simulink model "single_track_v2"  (R2024a)
settings: Solver=VariableStepAuto  StartTime=0.0  StopTime=145  RelTol=1e-3
undefined symbols (not defined in the file or in its folder): control_param, veh_param
libraries: simulink x5, autolibshared x1
settings Model: Creator=pair-andres  LastModifiedBy=pair-andres

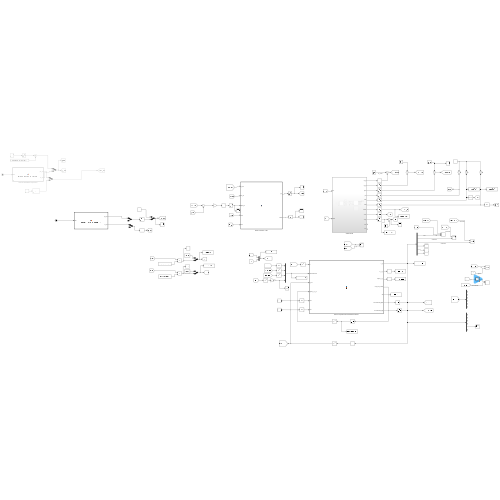
[thumbnail: Simulink's stored preview of the top-level diagram]
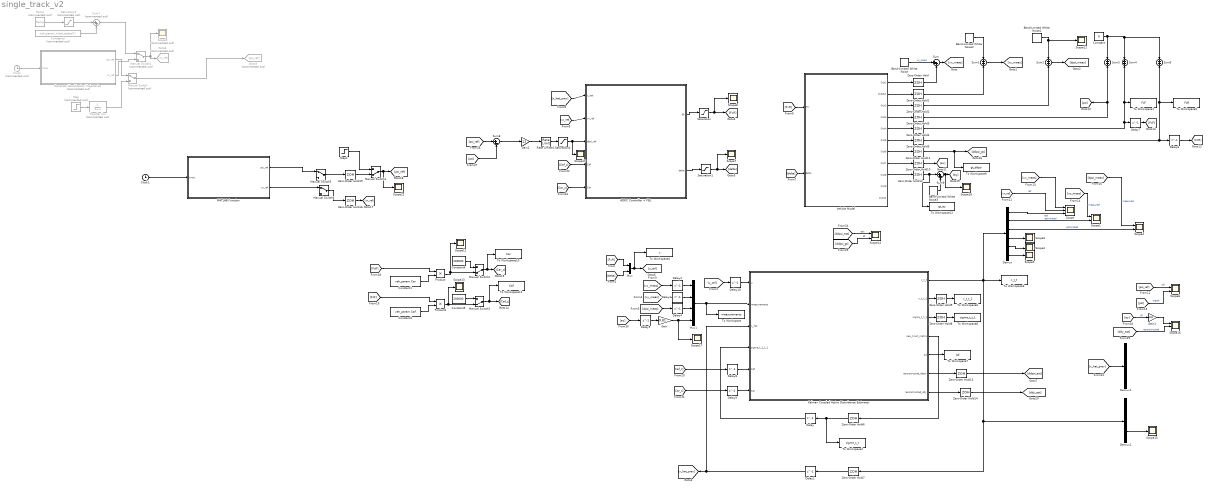
== system single_track_v2 ==
  ADRC Controller + FBL : MATLAB Function  TreatAsAtomicUnit=on
  Band-Limited White Noise : simulink/Sources/Band-Limited White Noise  Cov=[control_param.vx_noise_pwr]  Ts=control_param.T  seed=[23341]
  Band-Limited White Noise1 : simulink/Sources/Band-Limited White Noise  Cov=[control_param.dpsi_noise_pwr]  Ts=control_param.T  seed=[23343]
  Band-Limited White Noise2 : simulink/Sources/Band-Limited White Noise  Cov=[control_param.vy_noise_pwr]  Ts=control_param.T  seed=[23342]
  Band-Limited White Noise3 : simulink/Sources/Band-Limited White Noise  Cov=[control_param.dpsi_noise_pwr]  Ts=control_param.T  seed=[23343]
  Clock : Clock  Commented=on
  Clock1 : Clock
  Constant : Constant  Value=0
  Constant1 : Constant  Value=veh_param.Car  SampleTime=control_param.T
  Constant2 : Constant  Value=veh_param.Caf  SampleTime=control_param.T
  Constant3 : Constant  Commented=on  Value=veh_param.initial_states(1)
  Constant4 : Constant  Value=200000
  Constant5 : Constant  Value=200000
  Delay : Delay  DelayLength=1  InitialCondition=eye(6)*0  SampleTime=control_param.T
  Delay1 : Delay  DelayLength=1  InitialCondition=veh_param.initial_states  SampleTime=control_param.T
  Delay{2..5,8..10} (7 alike) : Delay  DelayLength=1  InitialCondition=0  SampleTime=control_param.T
  Delay6 : Delay  DelayLength=1  InitialCondition=veh_param.initial_states(1)  SampleTime=control_param.T
  Delay7 : Delay  DelayLength=1  InitialCondition=veh_param.initial_states(1)  SampleTime=control_param.T
  Demux : Demux  Outputs=6
  Demux1 : Demux  Outputs=6
  Demux2 : Demux  Outputs=6
  Gain : Gain  Gain=9.81
  Gain1 : Gain  Gain=9.81
  Gain2 : Gain  Gain=12
  Generate Identification Trajectories : MATLAB Function  Commented=on  TreatAsAtomicUnit=on
  Goto8 : Goto  Commented=on  GotoTag=vx_ref
  Goto9 : Goto  Commented=on  GotoTag=psi_ref
  Kalman Coupled Active Disturbance Estimator : MATLAB Function  TreatAsAtomicUnit=on
  MATLAB Function : MATLAB Function  TreatAsAtomicUnit=on
  Manual Switch : ManualSwitch  Commented=on
  Manual Switch1 : ManualSwitch  Commented=on
  Manual Switch2 : ManualSwitch  CurrentSetting=0
  Manual Switch3 : ManualSwitch  CurrentSetting=0
  Manual Switch4 : ManualSwitch  CurrentSetting=0
  Manual Switch5 : ManualSwitch
  Manual Switch6 : ManualSwitch
  Mux : Mux  Inputs=2
  Mux1 : Mux
  Product : Product
  Product1 : Product
  Ramp : simulink/Sources/Ramp  Commented=on  slope=5  start=2  InitialOutput=5
  Rate Limiter1 : RateLimiter  RisingSlewLimit=1.0  FallingSlewLimit=-1.0  SampleTimeMode=inherited
  Saturation : Saturate  UpperLimit=2000  LowerLimit=-4000
  Saturation1 : Saturate  UpperLimit=0.262  LowerLimit=-0.262
  Saturation2 : Saturate  Commented=on  UpperLimit=30
  Saturation4 : Saturate  UpperLimit=0.3  LowerLimit=-0.3
  Scope : Scope  NumInputPorts=3
  Scope{1..2,6,14} (4 alike) : Scope  NumInputPorts=2
  Scope{3..5,7..8,10..13,15,17..18,22} (13 alike) : Scope
  Scope16 : Scope  NumInputPorts=3
  Scope9 : Scope  Commented=on
  Step : Step  Commented=on  Time=5  After=0.1  SampleTime=0
  Step1 : Step  Time=0  After=0.05  SampleTime=control_param.T
  Sum : Sum  Inputs=|++
  Sum{1..5} (5 alike) : Sum
  Sum7 : Sum  Commented=on  Inputs=|++
  Sum8 : Sum  Inputs=|+-
  Sum9 : Sum  Inputs=|++
  To Workspace : ToWorkspace  VariableName=measurements  SaveFormat=Timeseries  SampleTime=control_param.T
  To Workspace1 : ToWorkspace  VariableName=FzF  SaveFormat=Timeseries  SampleTime=control_param.T
  To Workspace10 : ToWorkspace  VariableName=Car  SaveFormat=Timeseries  SampleTime=control_param.T
  To Workspace11 : ToWorkspace  VariableName=Caf  SaveFormat=Timeseries  SampleTime=control_param.T
  To Workspace12 : ToWorkspace  VariableName=gt_ay  SaveFormat=Timeseries  SampleTime=control_param.T
  To Workspace2 : ToWorkspace  VariableName=sigma_t_t  SaveFormat=Timeseries  SampleTime=0.01
      settings: Save2DSignal=2-D array (concatenate along first dimension)
  To Workspace3 : ToWorkspace  VariableName=x_t_t  SaveFormat=Timeseries  SampleTime=control_param.T
  To Workspace4 : ToWorkspace  VariableName=u  SaveFormat=Timeseries  SampleTime=control_param.T
  To Workspace5 : ToWorkspace  VariableName=FzR  SaveFormat=Timeseries  SampleTime=control_param.T
  To Workspace6 : ToWorkspace  VariableName=x_t_t_1  SaveFormat=Timeseries  SampleTime=0.01
  To Workspace7 : ToWorkspace  VariableName=Ad  SaveFormat=Timeseries  SampleTime=control_param.T
  To Workspace8 : ToWorkspace  VariableName=sigma_t_t_1  SaveFormat=Timeseries  SampleTime=0.01
      settings: Save2DSignal=2-D array (concatenate along first dimension)
  To Workspace9 : ToWorkspace  VariableName=gt_ddpsi  SaveFormat=Timeseries  SampleTime=control_param.T
  Transfer Fcn : TransferFcn  Commented=on  Denominator=[1 1]
  Vehicle Model : Subsystem
  Zero-Order Hold{,1..16} (17 alike) : ZeroOrderHold  SampleTime=control_param.T
  wires:
  Vehicle Model/2(Output) -> Zero-Order Hold1/1
  Constant/1 -> Sum5/1, Sum4/1, Sum3/1
  Sum/1 -> [vx_meas]
  Band-Limited White Noise2/1 -> Sum1/1
  Zero-Order Hold3/1 -> [psi], Sum3/2
  Zero-Order Hold4/1 -> Delay7/1, To Workspace1/1, Sum4/2
  Sum2/1 -> [dpsi_meas]
  Zero-Order Hold6/1 -> To Workspace2/1, Delay/1
  Band-Limited White Noise/1 -> Sum/1  "vx_noise"
  Zero-Order Hold1/1 -> Sum1/2
  Vehicle Model/6(Out5) -> Zero-Order Hold5/1
  Band-Limited White Noise1/1 -> Scope11/1, Sum2/1
  Vehicle Model/5(Out4) -> Zero-Order Hold4/1
  Delay/1 -> Kalman Coupled Active Disturbance Estimator/4(sigma_t_1_t_1)
  Vehicle Model/4(Out3) -> Zero-Order Hold3/1
  Vehicle Model/1(Out1) -> Zero-Order Hold/1
  Zero-Order Hold2/1 -> Sum2/2
  Vehicle Model/3(Out2) -> Zero-Order Hold2/1
  Sum1/1 -> [vy_meas]
  Zero-Order Hold/1 -> Sum/2
  Zero-Order Hold5/1 -> Delay6/1, To Workspace5/1, Sum5/2
  Kalman Coupled Active Disturbance Estimator/5(Ad) -> To Workspace7/1
  Kalman Coupled Active Disturbance Estimator/1(x_t_t) -> Demux2/1, Zero-Order Hold7/1, To Workspace3/1, Demux/1
  Zero-Order Hold7/1 -> Delay1/1
  Delay1/1 -> [x_hat_prev], Kalman Coupled Active Disturbance Estimator/3(x_hat)
  ADRC Controller + FBL/1(gp) -> Saturation/1
  ADRC Controller + FBL/2(delta) -> Saturation1/1
  [FxR] -> Mux/1
  [delta] -> Mux/2
  Mux/1 -> To Workspace4/1, [u_ctrl]
  Kalman Coupled Active Disturbance Estimator/2(x_t_t_1) -> Zero-Order Hold9/1
  Zero-Order Hold9/1 -> To Workspace6/1
  [u_ctrl] -> Delay10/1
  [dpsi_meas] -> Delay4/1
  [vx_meas] -> Delay2/1
  Mux1/1 -> To Workspace/1, Kalman Coupled Active Disturbance Estimator/2(measurements)
  [delta] -> Vehicle Model/2(delta)
  [FxR] -> Vehicle Model/1(Fxr)
  Kalman Coupled Active Disturbance Estimator/3(sigma_t_t_1) -> Zero-Order Hold8/1
  Zero-Order Hold8/1 -> To Workspace8/1
  Kalman Coupled Active Disturbance Estimator/4(new_trust_matrix) -> Zero-Order Hold6/1
  Kalman Coupled Active Disturbance Estimator/6(reconstructed_ddpsi) -> Zero-Order Hold13/1
  [x_hat_prev] -> ADRC Controller + FBL/1(x_hat)
  Clock/1 -> Generate Identification Trajectories/1(time)
  Demux/6 -> Scope5/1
  Demux/5 -> Scope4/1
  Demux/4 -> Scope3/1
  Demux/3 -> Scope2/2  "estimated"
  Demux/2 -> Scope1/2  "estimated"
  Demux/1 -> Scope/3  "est"
  [vx_ref] -> ADRC Controller + FBL/2(vx_ref)
  [vx_ref] -> Scope/2  "ref"
  Saturation/1 -> Scope8/1, [FxR]
  Saturation1/1 -> Scope7/1, [delta]
  [vx_meas] -> Scope/1
  [vy_meas] -> Scope1/1  "measured"
  Generate Identification Trajectories/1(psi_ref) -> Manual Switch/1
  Manual Switch/1 -> Goto9/1
  [psi_ref] -> Scope6/1  "ref"
  [psi] -> Scope6/2  "signal"
  [dpsi_meas] -> Scope2/1  "measured"
  Vehicle Model/8(Out7) -> Zero-Order Hold10/1
  Zero-Order Hold10/1 -> [ax]
  Step/1 -> Transfer Fcn/1
  Generate Identification Trajectories/2(vx_ref) -> Manual Switch1/2
  Manual Switch1/1 -> Goto8/1, Scope9/1
  Constant1/1 -> Product/2
  Constant2/1 -> Product1/2
  Product/1 -> Manual Switch2/2, Scope12/1
  Product1/1 -> Manual Switch3/2, Scope13/1
  [Car_z] -> Delay9/1
  [Caf_z] -> Delay8/1
  [Caf_z] -> ADRC Controller + FBL/4(Caf)
  [Car_z] -> ADRC Controller + FBL/5(Car)
  Ramp/1 -> Saturation2/1
  Constant3/1 -> Sum7/2
  Sum7/1 -> Manual Switch1/1
  Saturation2/1 -> Sum7/1
  [FzR] -> Product/1
  [FzF] -> Product1/1
  Vehicle Model/7(Out6) -> Zero-Order Hold11/1
  Zero-Order Hold11/1 -> To Workspace9/1, [ddpsi_gt]
  [ddpsi_est] -> Scope14/1  "est"
  [ddpsi_gt] -> Scope14/2  "gt"
  Constant4/1 -> Manual Switch2/1
  Constant5/1 -> Manual Switch3/1
  Transfer Fcn/1 -> Manual Switch/2
  Manual Switch2/1 -> To Workspace10/1, [Car_z]
  Manual Switch3/1 -> To Workspace11/1, [Caf_z]
  Step1/1 -> Manual Switch4/1
  Clock1/1 -> MATLAB Function/1(time)
  Manual Switch4/1 -> Scope22/1, [psi_ref]
  Gain2/1 -> Rate Limiter1/1
  Rate Limiter1/1 -> Saturation4/1
  [psi] -> Sum8/2
  [psi_ref] -> Sum8/1
  Saturation4/1 -> Scope10/1, ADRC Controller + FBL/3(dpsi_ref)
  Delay6/1 -> [FzR]
  Delay7/1 -> [FzF]
  [vy_meas] -> Delay3/1
  Vehicle Model/9(Out8) -> Zero-Order Hold12/1
  Kalman Coupled Active Disturbance Estimator/7(reconstructed_ddy) -> Zero-Order Hold14/1
  [ay] -> Gain1/1  "gt"
  [ddy_est] -> Scope16/2  "reconstructed"
  [ay] -> Delay5/1
  Zero-Order Hold12/1 -> To Workspace12/1, Sum9/1
  Band-Limited White Noise3/1 -> Sum9/2
  Sum9/1 -> Scope18/1, [ay]
  Sum8/1 -> Gain2/1
  Zero-Order Hold13/1 -> [ddpsi_est]
  Zero-Order Hold14/1 -> [ddy_est]
  [x_hat_prev] -> Demux1/1
  Delay2/1 -> Mux1/1
  Delay3/1 -> Mux1/2
  Delay4/1 -> Mux1/3
  Delay5/1 -> Gain/1
  Delay8/1 -> Kalman Coupled Active Disturbance Estimator/5(Caf)
  Delay9/1 -> Kalman Coupled Active Disturbance Estimator/6(Car)
  Delay10/1 -> Kalman Coupled Active Disturbance Estimator/1(u)
  Zero-Order Hold15/1 -> Manual Switch4/2
  Zero-Order Hold16/1 -> [vx_ref]
  Manual Switch5/1 -> Zero-Order Hold15/1
  MATLAB Function/1(psi_ref) -> Manual Switch5/1
  Manual Switch6/1 -> Zero-Order Hold16/1
  MATLAB Function/2(vx_ref) -> Manual Switch6/1
  Gain/1 -> Scope17/1, Mux1/4
  Demux2/5 -> Scope15/1
  Gain1/1 -> Scope16/1

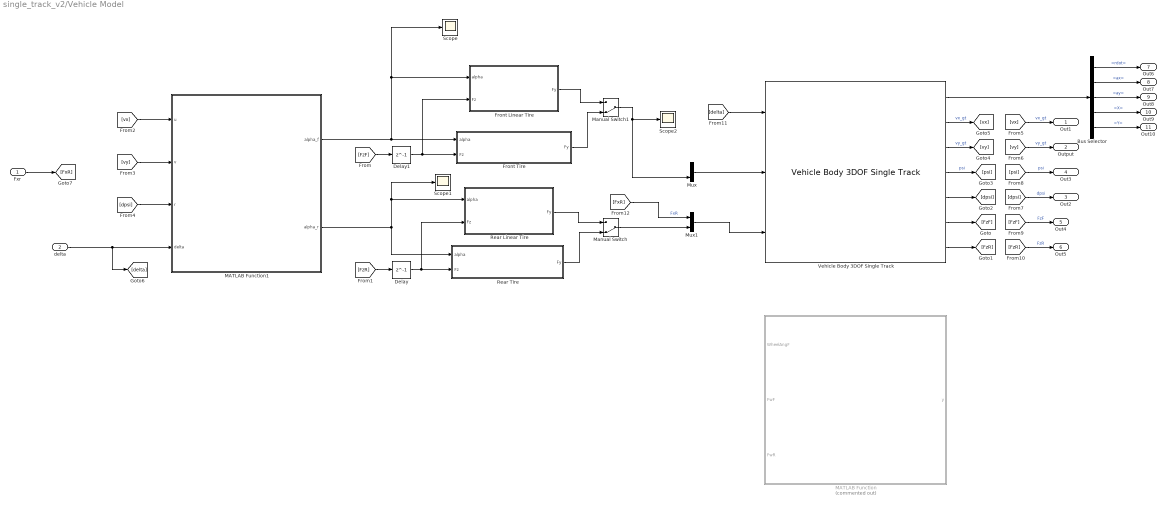
== system single_track_v2/Vehicle Model ==
  Fxr : Inport
  delta : Inport  Port=2
  Bus Selector : BusSelector  OutputSignals=BdyFrm.Cg.AngAcc.rdot,BdyFrm.Cg.Acc.ax,BdyFrm.Cg.Acc.ay,InertFrm.Cg.Disp.X,InertFrm.Cg.Disp.Y
  Delay : Delay  DelayLength=1  InitialCondition=veh_param.m*veh_param.g / 2  SampleTime=control_param.T
  Delay1 : Delay  DelayLength=1  InitialCondition=veh_param.m*veh_param.g / 2  SampleTime=control_param.T
  Front Linear Tire : MATLAB Function  TreatAsAtomicUnit=on
  Front Tire : MATLAB Function  TreatAsAtomicUnit=on
  MATLAB Function : MATLAB Function  Commented=on  TreatAsAtomicUnit=on
  MATLAB Function1 : MATLAB Function  TreatAsAtomicUnit=on
  Manual Switch : ManualSwitch  CurrentSetting=0
  Manual Switch1 : ManualSwitch  CurrentSetting=0
  Mux : Mux  Inputs=2
  Mux1 : Mux  Inputs=2
  Rear Linear Tire : MATLAB Function  TreatAsAtomicUnit=on
  Rear Tire : MATLAB Function  TreatAsAtomicUnit=on
  Scope : Scope
  Scope1 : Scope
  Scope2 : Scope
  Vehicle Body 3DOF Single Track : autolibshared/Vehicle Body 3DOF Single Track  trackMode=Single (bicycle)  inputMode=External forces  frontSteerMode=on  rearSteerMode=off  windMode=off  muMode=off  extFMode=off  extMMode=off  htchFMode=off  htchMMode=off  extXo=off  extpsio=off  extxdoto=off  extro=off  extYo=off  extTamb=off  extydoto=off  aMode=2  NF=2  NR=2  m=veh_param.m  a=veh_param.lf  b=veh_param.lr  h=0.35  dh=1  hh=0.2  X_o=0  xdot_o=veh_param.initial_states(1)  CalphaMode=off  sigmaMode=on  d=0  hl=0  w=[1.4,1.4]  Cy_f=12e3  Cy_r=11e3  sigma_f=.1  sigma_r=.1  alpha_f_brk=[-.1 .1]  Cy_f_data=[-9e3 9e3]  alpha_r_brk=[-.1 .1]  Cy_r_data=[-9e3 9e3]  Y_o=500  ydot_o=0  Izz=1000  psi_o=0  r_o=0  Af=2.0  Cd=veh_param.Cd  Cl=.1  Cpm=.1  beta_w=[0 0.01:0.01:0.3]  Cs=[0 0.01:0.01:0.3]  Cym=[0 1e-6:0.01:0.3]  Pabs=101325  Tair=273  g=9.81  mu=1  xdot_tol=.01  Fznom=5000  Fxtire_sat=7e4  Fytire_sat=7e4  longOff=0  latOff=0  vertOff=0  wrapAng=off
  Out1 : Outport
  Output : Outport  Port=2
  Out2 : Outport  Port=3
  Out3 : Outport  Port=4
  Out4 : Outport  Port=5
  Out5 : Outport  Port=6
  Out6 : Outport  Port=7
  Out7 : Outport  Port=8
  Out8 : Outport  Port=9
  Out9 : Outport  Port=10
  Out10 : Outport  Port=11
  wires:
  Bus Selector/5 -> Out10/1  "<Y>"
  Bus Selector/2 -> Out7/1  "<ax>"
  [FzF] -> Delay1/1
  Vehicle Body 3DOF Single Track/3 -> [vy]  "vy_gt"
  Mux/1 -> Vehicle Body 3DOF Single Track/2
  Vehicle Body 3DOF Single Track/1 -> Bus Selector/1
  Bus Selector/1 -> Out6/1  "<rdot>"
  [FzR] -> Out5/1  "FzR"
  Vehicle Body 3DOF Single Track/4 -> [psi]  "psi"
  [vx] -> MATLAB Function1/1(u)
  Fxr/1 -> [FxR]
  MATLAB Function1/2(alpha_r) -> Scope1/1, Rear Linear Tire/1(alpha), Rear Tire/1(alpha)
  Vehicle Body 3DOF Single Track/7 -> [FzR]
  Rear Linear Tire/1(Fy) -> Manual Switch/1
  [FzR] -> Delay/1
  Vehicle Body 3DOF Single Track/5 -> [dpsi]
  MATLAB Function1/1(alpha_f) -> Scope/1, Front Linear Tire/1(alpha), Front Tire/1(alpha)
  Bus Selector/4 -> Out9/1  "<X>"
  Vehicle Body 3DOF Single Track/6 -> [FzF]
  Vehicle Body 3DOF Single Track/2 -> [vx]  "vx_gt"
  [vy] -> MATLAB Function1/2(v)
  [dpsi] -> Out2/1  "dpsi"
  Mux1/1 -> Vehicle Body 3DOF Single Track/3
  [delta] -> Vehicle Body 3DOF Single Track/1
  delta/1 -> [delta], MATLAB Function1/4(delta)
  Rear Tire/1(Fy) -> Manual Switch/2
  Front Tire/1(Fy) -> Manual Switch1/2
  Front Linear Tire/1(Fy) -> Manual Switch1/1
  [dpsi] -> MATLAB Function1/3(r)
  Bus Selector/3 -> Out8/1  "<ay>"
  [FxR] -> Mux1/1  "FxR"
  [psi] -> Out3/1  "psi"
  [FzF] -> Out4/1  "FzF"
  [vx] -> Out1/1  "vx_gt"
  [vy] -> Output/1  "vy_gt"
  Delay/1 -> Rear Linear Tire/2(Fz), Rear Tire/2(Fz)
  Delay1/1 -> Front Linear Tire/2(Fz), Front Tire/2(Fz)
  Manual Switch/1 -> Mux1/2
  Manual Switch1/1 -> Scope2/1, Mux/2

== matlab function single_track_v2/Vehicle Model/MATLAB Function1 ==
  data: u input; alpha_f output; v input; r input; delta input; alpha_r output; veh_param parameter
function [alpha_f, alpha_r] = calc_bicycle_slip_angles(u, v, r, delta, veh_param)
% Calculate slip angles at the tires:
% WARNING: Careful with sign conventions used in the model, make sure you
% get this right

lf = veh_param.lf;
lr = veh_param.lr;


theta_v_f = atan2(v + r * lf, u);

theta_v_r = atan2(v - r * lr, u);

% Front: Steer angle is delta, velocity angle is theta_v_f
alpha_f = theta_v_f - delta;

% Rear: Steer angle is 0, velocity angle is theta_v_r
alpha_r = theta_v_r;

end

== matlab function single_track_v2/Vehicle Model/Rear Linear Tire ==
  data: alpha input; Fy output; Fz input; veh_param parameter
function Fy = linear_tire_model(alpha, Fz, veh_param)
    % Implements a simple LINEAR tire model.
    %
    % Fy = C_alpha * alpha
    %
    % To be a fair comparison to your Pacejka block, we define
    % C_alpha as the initial slope of the Pacejka curve, which
    % is load-dependent.
    
    % TIRE PACEJKA PARAMS:
    B = veh_param.Br;
    C = veh_param.Cr;
    D = veh_param.Dr;
    E = veh_param.Er;
    
    % The linear cornering stiffness (C_alpha) for small angles
    % is the product of B, C, and D, scaled by Fz.
    % K is the "cornering stiffness coefficient".
    K_pacejka = B * C * D; % 22 * 1.8 * 1.6 = 63.36
    
    % --- Safety Check: Ensure Fz is positive ---
    Fz_pos = max(0, Fz);
    
    % --- 1. Calculate Cornering Stiffness ---
    C_alpha = K_pacejka * Fz_pos; % K * Fz_pos;
    
    % --- 2. Linear Force Calculation ---
    Fy = C_alpha * alpha;
end

== matlab function single_track_v2/Vehicle Model/Rear Tire ==
  data: alpha input; Fy output; Fz input; veh_param parameter
function Fy = simple_pacejka_lat(alpha, Fz, veh_param)

    % Implements the simple Pacejka '89 lateral force model.
    %
    % INPUTS:
    %   alpha:  Tire Slip Angle (radians)
    %   Fz:     Vertical Load on the tire (Newtons)
    %
    % OUTPUT:
    %   Fy:     Lateral Force (Newtons)
    
    % TIRE PACEJKA PARAMS:
    %   B:      Stiffness Factor
    %   C:      Shape Factor
    %   D:      Peak Factor (Peak friction coefficient, mu_y)
    %   E:      Curvature Factor
       
    % Front tire pacejka parameters:
    B = veh_param.Br;
    C = veh_param.Cr;
    D = veh_param.Dr;
    E = veh_param.Er;
    
    % --- Safety Check: Ensure Fz is positive ---
    % The formula assumes positive vertical load.
    Fz_pos = max(0, Fz);
    
    % --- 1. Calculate Peak Lateral Force ---
    % D is the friction coefficient, so F_peak = D * Fz
    F_peak = D * Fz_pos;
    
    % --- 2. Composite Slip Term ---
    % This is the main input to the sine function
    x = B * alpha;
    
    % --- 3. Pacejka '89 "Magic Formula" ---
    % This is the core equation
    Fy = -F_peak * sin(C * atan(x - E * (x - atan(x))));

end

== matlab function single_track_v2/Generate Identification Trajectories ==
  data: psi_ref output; vx_ref output; time input
function [psi_ref, vx_ref] = generate_identification_trajectory(time)
%#codegen
% Generates feasible, persistently exciting reference signals for 
% Vehicle System Identification.
%
% INPUT:
%   time: Current simulation time (seconds)
%
% OUTPUTS:
%   psi_ref: Global heading reference (radians)
%   vx_ref:  Longitudinal velocity reference (m/s) [10 to 40 m/s]
    

    % --- CONFIGURATION ---
    TEST_DURATION = 150; % Total test time (seconds)
    
    % Velocity Constraints
    V_MIN = 10; % m/s
    V_MAX = 40; % m/s
    
    % Heading Chirp Parameters
    % We want to sweep from gentle turns to aggressive slalom
    FREQ_START = 0.1; % Hz (Slow turns)
    FREQ_END   = 0.8; % Hz (Fast slalom - verify your sampling rate > 2*FREQ_END)
    AMP_YAW    = 0.1; % rad (Approx 30 degrees max heading deviation)

    % --- 1. GENERATE VELOCITY REFERENCE (vx_ref) ---
    % We use a slow sine wave to sweep through the speed range.
    % This ensures we test high-speed/low-steer and low-speed/high-steer.
    
    % Period of speed change (make it slower than steering dynamics)
    v_period = 10; 
    
    % Sine wave scaled to [V_MIN, V_MAX]
    % 0.5*(Max-Min)*sin(...) + 0.5*(Max+Min)
    vx_ref = 0.5 * (V_MAX - V_MIN) * sin(2 * pi * (1/v_period) * time - pi/2) ...
           + 0.5 * (V_MAX + V_MIN);
       
    % Clamp for safety (redundant but good practice)
    if vx_ref < V_MIN; vx_ref = V_MIN; end
    if vx_ref > V_MAX; vx_ref = V_MAX; end

    % --- 2. GENERATE HEADING REFERENCE (psi_ref) ---
    % We use a "Chirp" signal (Swept Sine) for the heading.
    % Ideally, we want the yaw rate to be the chirp, so psi is the integral.
    
    if time < 10
        % Stop the test
        psi_ref = 0;
        vx_ref = 5;

    elseif time <= TEST_DURATION
        % Instantaneous frequency f(t) = f0 + k*t
        k = (FREQ_END - FREQ_START) / TEST_DURATION;
        
        % Phase = integral of frequency
        % phi(t) = 2*pi * (f0*t + 0.5*k*t^2)
        phase = 2 * pi * (FREQ_START * time + 0.5 * k * time^2*0.2);
        
        % We modulate the amplitude based on speed to keep lateral accel safe-ish.
        % At 40 m/s, we can't turn as sharp as at 10 m/s.
        % Scaling factor: inversely proportional to speed
        safe_scaling = (V_MIN / vx_ref); 
        
        % The Heading Reference
        psi_ref = (AMP_YAW * safe_scaling) * sin(phase);
    else
        psi_ref = 0;
        vx_ref = 0;
    end
end

== matlab function single_track_v2/MATLAB Function ==
  data: time input; psi_ref output; vx_ref output
function [psi_ref, vx_ref] = generate_identification_trajectory(time)
%#codegen
% Generates feasible, persistently exciting reference signals for 
% Vehicle System Identification.
%
% INPUT:
%   time: Current simulation time (seconds)
%
% OUTPUTS:
%   psi_ref: Global heading reference (radians)
%   vx_ref:  Longitudinal velocity reference (m/s) [10 to 40 m/s]

    % --- CONFIGURATION ---
    TEST_DURATION = 150; % Total test time (seconds)
    
    % Velocity Constraints
    V_MIN = 10; % m/s
    V_MAX = 80; % m/s
    
    % Heading Chirp Parameters
    % We want to sweep from gentle turns to aggressive slalom
    FREQ_START = 0.001; % Hz (Slow turns)
    FREQ_END   = 0.8; % Hz (Fast slalom - verify your sampling rate > 2*FREQ_END)
    AMP_YAW    = 0.35; % rad (Approx 30 degrees max heading deviation)

    % --- 1. GENERATE VELOCITY REFERENCE (vx_ref) ---
    % We use a slow sine wave to sweep through the speed range.
    % This ensures we test high-speed/low-steer and low-speed/high-steer.
    
    % Period of speed change (make it slower than steering dynamics)
    v_period = 100; 
    
    % Sine wave scaled to [V_MIN, V_MAX]
    % 0.5*(Max-Min)*sin(...) + 0.5*(Max+Min)
    vx_ref = 0.5 * (V_MAX - V_MIN) * sin(2 * pi * (1/v_period) * time - pi/2) ...
           + 0.5 * (V_MAX + V_MIN);
       
    % Clamp for safety (redundant but good practice)
    if vx_ref < V_MIN; vx_ref = V_MIN; end
    if vx_ref > V_MAX; vx_ref = V_MAX; end

    % --- 2. GENERATE HEADING REFERENCE (psi_ref) ---
    % We use a "Chirp" signal (Swept Sine) for the heading.
    % Ideally, we want the yaw rate to be the chirp, so psi is the integral.
    
    if time <= TEST_DURATION
        % Instantaneous frequency f(t) = f0 + k*t
        k = (FREQ_END - FREQ_START) / TEST_DURATION;
        
        % Phase = integral of frequency
        % phi(t) = 2*pi * (f0*t + 0.5*k*t^2)
        phase = 2 * pi * (FREQ_START * time + 0.5 * k * time^2*0.2);
        
        % We modulate the amplitude based on speed to keep lateral accel safe-ish.
        % At 40 m/s, we can't turn as sharp as at 10 m/s.
        % Scaling factor: inversely proportional to speed
        safe_scaling = (V_MIN / vx_ref); 
        
        % The Heading Reference
        psi_ref = (AMP_YAW * safe_scaling) * sin(phase);
    else
        % Stop the test
        psi_ref = 0;
        vx_ref = 0;
    end
end

== matlab function single_track_v2/Vehicle Model/MATLAB Function ==
  data: WheelAngF input; y output; FwF input; FwR input
function y = fcn(WheelAngF, FwF, FwR)

y = u;

== matlab function single_track_v2/ADRC Controller + FBL ==
  data: gp output; x_hat input; vx_ref input; dpsi_ref input; delta output size=[1]; control_param parameter; veh_param parameter; Caf input; Car input
function [gp, delta] = fcn(x_hat, vx_ref, dpsi_ref, control_param, veh_param, Caf, Car)
% Implements a model-based ADRC controller by actively canceling
% the known linear vehicle dynamics and the estimated disturbance.

% --- 1. Unpack State Vector ---
% We assume the state vector is: x_hat = [vx, vy, r, xi_x, xi_y, xi_psi]'
DECCEL_THRESHOLD = control_param.deccel_threshold;

dx   = x_hat(1); % vx (forward velocity)
dy   = x_hat(2); % vy (lateral velocity)
dpsi = x_hat(3); % r  (yaw rate)
xi_hat_x   = x_hat(4); % Estimated x-disturbance
xi_hat_y   = x_hat(5); % Estimated y-disturbance
xi_hat_psi = x_hat(6); % Estimated psi-disturbance

% Caf = veh_param.Caf * veh_param.m * veh_param.g / 2; % NOTE: We are not modeling load transfer on this linear model, but estimated is mass/2 supported
% Car = veh_param.Car * veh_param.m * veh_param.g / 2; % NOTE: We are not modeling load transfer on this linear model, but estimated is mass/2 supported

Izz = veh_param.Izz;
m = veh_param.m;
lf = veh_param.lf;
lr = veh_param.lr;
Cd = veh_param.Cd;
K1l = control_param.K1_vx;
K1 = control_param.K1_dpsi; 

% --- 2. Longitudinal Control (gp) ---
% Model: m*dvx = gp + xi_x
% This controller cancels the disturbance and applies a P-controller
% on velocity error.
U0_x = K1l*(vx_ref - dx) - (xi_hat_x / m) + Cd*dx/m;
Fdesired = m * U0_x;

% 2.2. Apply Deadband Logic
if Fdesired > 0
    % The command is positive, so we apply throttle.
    gp = Fdesired;
elseif -Fdesired/m > DECCEL_THRESHOLD
    % The command is negative AND has exceeded our "coasting" threshold.
    % We apply the brakes.
    gp = Fdesired;
else
    % The command is slightly negative (e.g., -10N).
    % This is inside the deadband, so we just coast.
    gp = 0;
end



% --- 3. Lateral/Yaw Control (delta) ---
% This is the new, model-based ADRC.

% 3.1. Calculate linear coupling terms (Nv, Nr)
% These are the terms of 'A_aug' matrix that couple vy and r.
% (We add a small epsilon to dx to avoid division by zero if the car stops)
vx = dx + 1e-6; 
Nv = -(Caf*lf - Car*lr) / (Izz * vx);
Nr = -(Caf*lf^2 + Car*lr^2) / (Izz * vx);

% 3.2. Define the "virtual control" (U0_psi)
% This is the total yaw acceleration we want to command.
% U0_psi = (Reference Accel) + (PD Control) - (Linear Feedback) - (Disturbance Feedback)

psi_ddot_ref = 0; % Assuming reference yaw acceleration is 0 for path following

linear_feedback = (Nv * dy + Nr * dpsi);
disturbance_feedback = (xi_hat_psi / Izz);
pd_control = K1*(dpsi_ref - dpsi); % Your P-controller on rate error

U0_psi = psi_ddot_ref + pd_control - linear_feedback - disturbance_feedback;

% 3.3. Invert the linear control model (B_lin) to find delta
% Our linear model's control input part is: ddot_psi = ... + (2*Caf*lf / Izz) * delta
% We set U0_psi equal to this known control part and solve for delta.
B_lin_psi = (Caf*lf) / Izz;
delta = U0_psi / B_lin_psi;

% Saturation added outside in Smulink

end

== matlab function single_track_v2/Kalman Coupled Active Disturbance Estimator ==
  data: u input; x_t_t output; x_t_t_1 output; sigma_t_t_1 output; measurements input; x_hat input; sigma_t_1_t_1 input; new_trust_matrix output; Ad output; reconstructed_ddpsi output; veh_param parameter; control_param parameter; Caf input; Car input; reconstructed_ddy output
function [x_t_t, x_t_t_1, sigma_t_t_1, new_trust_matrix, Ad, reconstructed_ddpsi, reconstructed_ddy]= fcn(u, measurements, x_hat, sigma_t_1_t_1, veh_param, control_param, Caf, Car)

T = control_param.T; % seconds

% var = vx_noise_power / T
R_vx = control_param.ekf_vx_sensor_noise;   
R_vy = control_param.ekf_vy_sensor_noise; 
R_dpsi = control_param.ekf_dpsi_sensor_noise; 
R_ay = control_param.ekf_ay_sensor_noise;

% Sensor noise:
% vx_noise_power = control_param.vx_noise_pwr;
% vy_noise_power = control_param.vy_noise_pwr;
% dpsi_noise_power = control_param.dpsi_noise_pwr;

% Variances for each state: [vx, vy, r, xi_x, xi_y, xi_psi]
Q_diag = control_param.ekf_Q_diag;


sigma_y_given_x = diag([R_vx, R_vy, R_dpsi, R_ay]);
sigma_x = diag(Q_diag);


% Vehicle parameters:
lf = veh_param.lf; lr = veh_param.lr;
m = veh_param.m; 
Izz = veh_param.Izz;
Cd = veh_param.Cd;


vx = x_hat(1);  %dx



% Linear Bicycle Model Terms
Yv = -(Caf + Car) / (m * max(vx, 1));
Yr = -vx - (Caf*lf - Car*lr) / (m * max(vx, 1));
Nv = -(Caf*lf - Car*lr) / (Izz * max(vx, 1));
Nr = -(Caf*lf^2 + Car*lr^2) / (Izz * max(vx, 1));

% Build the new, physically-correct A_aug matrix
% We assume vx dynamics are separate (e.g., dvx = 1/m * Fx_input + 1/m * xi_x)
A_aug = [
    -Cd/m,   0,   0,   1/m,   0,     0;     % dvx equation (no coupling)
    0,   Yv,  Yr,  0,     1/m,   0;     % dvy equation (COUPLED)
    0,   Nv,  Nr,  0,     0,     1/Izz; % dr equation (COUPLED)
    0,   0,   0,   0,     0,     0;     % d(xi_x)
    0,   0,   0,   0,     0,     0;     % d(xi_y)
    0,   0,   0,   0,     0,     0      % d(xi_psi)
];

C_aug = [
   eye(3), zeros(3);
   0, Yv, Yr + vx,  0, 1/m, 0;    % Computes ay (NEW) % Yr + vx
];




% Build matrix B which depends on state variables and complicated terms:

% b21 = 0;
% b22 = (1/m) * (2*Caf*dx/(dx+dy+dpsi*lf));
% 
% b41 = 0;
% b42 = (1/Izz) * (2*lf*Caf*dx/(dx+dy+dpsi*lf));

B_aug = [
    1/m, 0;
    0, Caf/m;
    0, Caf*lf/Izz;
    0, 0;
    0, 0;
    0, 0
];

% Discretize state-space with Zero Order Hold (ZOH):
Ad = eye(6) + A_aug*T;
Bd = T*B_aug;
% Note Caug is already our Cdiscrete

% disp('vx')
% disp(dx)


% Predict (Time Update):
x_t_t_1 = Ad*x_hat + Bd*u;
sigma_t_t_1 = Ad * sigma_t_1_t_1 * Ad' + sigma_x;



% Update (Measurement Update):
Kt = sigma_t_t_1 * C_aug' * inv(C_aug*sigma_t_t_1*C_aug' + sigma_y_given_x);
x_t_t = x_t_t_1 + Kt * (measurements - C_aug*x_t_t_1);

% sigma_t_t = sigma_t_t_1 - Kt * C_aug * sigma_t_t_1;
I = eye(6);
% sigma_t_t = (I - Kt * C_aug) * sigma_t_t_1;
sigma_t_t = (I - Kt*C_aug) * sigma_t_t_1 * (I - Kt*C_aug)' + Kt*sigma_y_given_x*Kt';



new_trust_matrix = sigma_t_t;



% Build disturbances can we?
psi_ddot_lin = (Nv * x_t_t(2) + Nr * x_t_t(3)) + B_aug(3,2)*u(2);%+ (Caf*lf* u(2)/Izz);

psi_ddot_disturbance = x_t_t(6) / Izz;

% disp('x_t_t(2)*Yv');
% disp(x_t_t(2)*Yv);
% 
% disp('x_t_t(3)*Yr');
% disp(Yr*x_t_t(3));
% 
% disp('B_aug(2,2)*u(2)');
% disp(B_aug(2,2)*u(2));
% 
% disp('x_t_t(5)/m');
% disp(x_t_t(5)/m);


y_ddot_adrc = Yv*x_t_t(2) + Yr*x_t_t(3) + B_aug(2,2)*0*u(2) + x_t_t(5)/m;

reconstructed_ddy = y_ddot_adrc + x_t_t(1)*x_t_t(3); % IMU gives us ddy

reconstructed_ddpsi = psi_ddot_lin + psi_ddot_disturbance;

% xi_psi_analytic = (-(2*lf*Caf*(dy+dpsi*lf)*cos(u(2)))/(dx+dy+dpsi*lf) + (2*lr*Car*(dy-dpsi*lf))/(dx) ) *(1/Izz);

== matlab function single_track_v2/Vehicle Model/Front Linear Tire ==
  data: alpha input; Fy output; Fz input; veh_param parameter
function Fy = linear_tire_model(alpha, Fz, veh_param)
    % Implements a simple LINEAR tire model.
    %
    % Fy = C_alpha * alpha
    
    B = veh_param.Bf;
    C = veh_param.Cf;
    D = veh_param.Df;

    % The linear cornering stiffness (C_alpha) for small angles
    % is the product of B, C, and D, scaled by Fz.
    % K is the "cornering stiffness coefficient".
    K_pacejka = B * C * D; % 22 * 1.8 * 1.6 = 63.36
    
    % --- Safety Check: Ensure Fz is positive ---
    Fz_pos = max(0, Fz);
    
    % --- 1. Calculate Cornering Stiffness ---
    C_alpha = K_pacejka * Fz_pos; % K * Fz_pos;
    
    % --- 2. Linear Force Calculation ---
    Fy = C_alpha * alpha;
end

== matlab function single_track_v2/Vehicle Model/Front Tire ==
  data: alpha input; Fy output; Fz input; veh_param parameter
function Fy = simple_pacejka_lat(alpha, Fz, veh_param)

    % Implements the simple Pacejka '89 lateral force model.
    %
    % INPUTS:
    %   alpha:  Tire Slip Angle (radians)
    %   Fz:     Vertical Load on the tire (Newtons)
    %
    % OUTPUT:
    %   Fy:     Lateral Force (Newtons)

    % TIRE PACEJKA PARAMS:
    %   B:      Stiffness Factor
    %   C:      Shape Factor
    %   D:      Peak Factor (Peak friction coefficient, mu_y)
    %   E:      Curvature Factor
    
    % Front tire pcejka parameters:
    B = veh_param.Bf;
    C = veh_param.Cf;
    D = veh_param.Df;
    E = veh_param.Ef;

    
    % --- Safety Check: Ensure Fz is positive ---
    % The formula assumes positive vertical load.
    Fz_pos = max(0, Fz);
    
    % --- 1. Calculate Peak Lateral Force ---
    % D is the friction coefficient, so F_peak = D * Fz
    F_peak = D * Fz_pos;
    
    % --- 2. Composite Slip Term ---
    % This is the main input to the sine function
    x = B * alpha;
    
    % --- 3. Pacejka '89 "Magic Formula" ---
    % This is the core equation
    Fy = -F_peak * sin(C * atan(x - E * (x - atan(x))));

end
